simulink model "model"  (R2024a)
settings: Solver=VariableStepAuto  StartTime=0.0  StopTime=0.2  RelTol=1e-3
libraries: dspfdesign x1
settings Model: Creator=hares  LastModifiedBy=hares

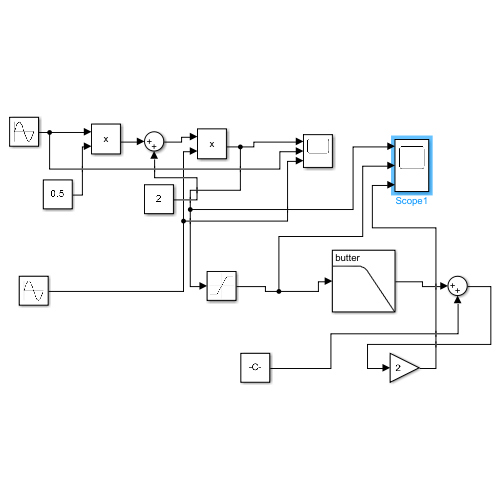
[thumbnail: Simulink's stored preview of the top-level diagram]
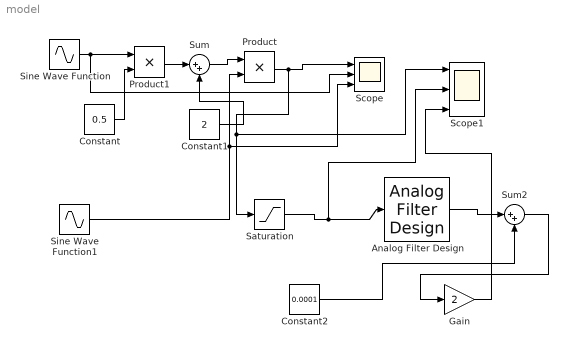
== system model ==
  Analog Filter Design : dspfdesign/Analog Filter Design  method=Butterworth  filttype=Lowpass  N=4  Wlo=100  Whi=80  Rp=2  Rs=40
  Constant : Constant  Value=0.5
  Constant1 : Constant  Value=2
  Constant2 : Constant  Value=0.0001
  Gain : Gain  Gain=2
  Product : Product
  Product1 : Product
  Saturation : Saturate  UpperLimit=5  LowerLimit=0
  Scope : Scope  NumInputPorts=3
  Scope1 : Scope  NumInputPorts=3
  Sine Wave Function : Sin  Amplitude=2  Frequency=100  Phase=3.14  SampleTime=0
  Sine Wave Function1 : Sin  Amplitude=2  Frequency=1000  Phase=3.14  SampleTime=0
  Sum : Sum  Inputs=|++
  Sum2 : Sum  Inputs=|++
  wires:
  Sine Wave Function/1 -> Scope/2, Product1/1
  Constant/1 -> Product1/2
  Product1/1 -> Sum/1
  Constant1/1 -> Sum/2
  Sum/1 -> Product/1
  Sine Wave Function1/1 -> Scope/3, Product/2
  Product/1 -> Saturation/1, Scope1/1, Scope/1
  Saturation/1 -> Scope1/2, Analog Filter Design/1
  Analog Filter Design/1 -> Sum2/1
  Constant2/1 -> Sum2/2
  Sum2/1 -> Gain/1
  Gain/1 -> Scope1/3
